simulink model "sldemo_bus_arrays"  (Simulink 10.0)
settings: Solver=FixedStepDiscrete  StartTime=0.0  StopTime=10  FixedStep=0.2  RelTol=1e-3  EnableMultiTasking=on
PreLoadFcn:
  | load sldemo_bus_arrays_data.mat;
undefined symbols (not defined in the file): a, b
Description:
  | Modeling Arrays of Buses
  | 
  | This example illustrates the use of arrays of buses in Simulink(R) to represent structured data compactly, eliminating the need to include multiple copies of the same buses.You can also use For Each subsystems to iteratively process each element of the bus array.
  | 
  | In this example, the array of buses is created using a Vector Concatenate block. The input bus signals to the Concatenate block must be nonvirtual and of the same type (that is, have the same names, hierarchies and attributes for the leaf elements).
  | 
  | The example also illustrates the use of the Selector and Assignment blocks to select from and assign into the array of buses.
CloseFcn:
  | evalin('base', 'clear sldemo_bus_arrays_busobject;');
settings Model: Creator=The MathWorks, Inc.  LastModifiedBy=bhisma
settings DataIOCC: LimitDataPoints=on  SaveFormat=StructureWithTime  SaveOutput=off  SaveTime=off  ReturnWorkspaceOutputs=on
settings OptimizationCC: BlockReduction=off  OptimizeBlockIOStorage=off  BufferReuse=off  GlobalBufferReuse=off  ExpressionFolding=off  PassReuseOutputArgsAs=Individual arguments  ExpressionDepthLimit=2147483647  LocalBlockOutputs=off  EfficientFloat2IntCast=on  OptimizeDataStoreBuffers=off  BusAssignmentInplaceUpdate=off  EfficientTunableParamExpr=on
settings DebuggingCC: ConsistencyChecking=warning  SignalInfNanChecking=error  SignalRangeChecking=error  ReadBeforeWriteMsg=EnableAllAsError  WriteAfterWriteMsg=EnableAllAsError  WriteAfterReadMsg=EnableAllAsError  AlgebraicLoopMsg=error  SaveWithDisabledLinksMsg=error  SaveWithParameterizedLinksMsg=error  UnderspecifiedInitializationDetection=Simplified  MergeDetectMultiDrivingBlocksExec=error  CheckExecutionContextPreStartOutputMsg=on  CheckExecutionContextRuntimeOutputMsg=on  BlockPriorityViolationMsg=error  SolverPrmCheckMsg=error  InheritedTsInSrcMsg=error  SigSpecEnsureSampleTimeMsg=error  CheckMatrixSingularityMsg=error  IntegerOverflowMsg=error  ParameterUnderflowMsg=error  ParameterPrecisionLossMsg=error  ParameterTunabilityLossMsg=error  UnderSpecifiedDataTypeMsg=error  UnnecessaryDatatypeConvMsg=warning  VectorMatrixConversionMsg=error  FcnCallInpInsideContextMsg=warning  SignalLabelMismatchMsg=error  UnconnectedInputMsg=error  UnconnectedOutputMsg=error  UnconnectedLineMsg=error  SFcnCompatibilityMsg=error  BusObjectLabelMismatch=error  RootOutportRequireBusObject=error  AssertControl=DisableAll  ModelReferenceIOMsg=error  ModelReferenceVersionMismatchMessage=error  ModelReferenceIOMismatchMessage=error  UnknownTsInhSupMsg=error  ModelReferenceDataLoggingMessage=error  StateNameClashWarn=warning  StrictBusMsg=ErrorOnBusTreatedAsVector  IntegerSaturationMsg=error
settings SFSimCC: MATLABDynamicMemAlloc=off
settings RTWCC: Description=Real-Time Workshop Embedded Coder  SystemTargetFile=ert.tlc  GenCodeOnly=on  TemplateMakefile=ert_default_tmf  GenerateReport=on  IncludeHyperlinkInReport=on  LaunchReport=on
settings CodeAppCC: ForceParamTrailComments=on  IgnoreCustomStorageClasses=off  MangleLength=4  CustomSymbolStrType=$N$R$M  InternalIdentifier=Classic  ReqsInCode=on
settings ERTTargetCC: MultiwordLength=2048  GenerateSampleERTMain=on  IncludeMdlTerminateFcn=off  GeneratePreprocessorConditionals=Disable all  SuppressErrorStatus=on  SupportAbsoluteTime=off  SupportNonFinite=off  ParenthesesLevel=Maximum  ERTCustomFileTemplate=example_file_process.tlc  PreserveExpressionOrder=on  PreserveIfCondition=on  ConvertIfToSwitch=off  SuppressUnreachableDefaultCases=off
settings ConfigComp: CovExternalEMLEnable=off

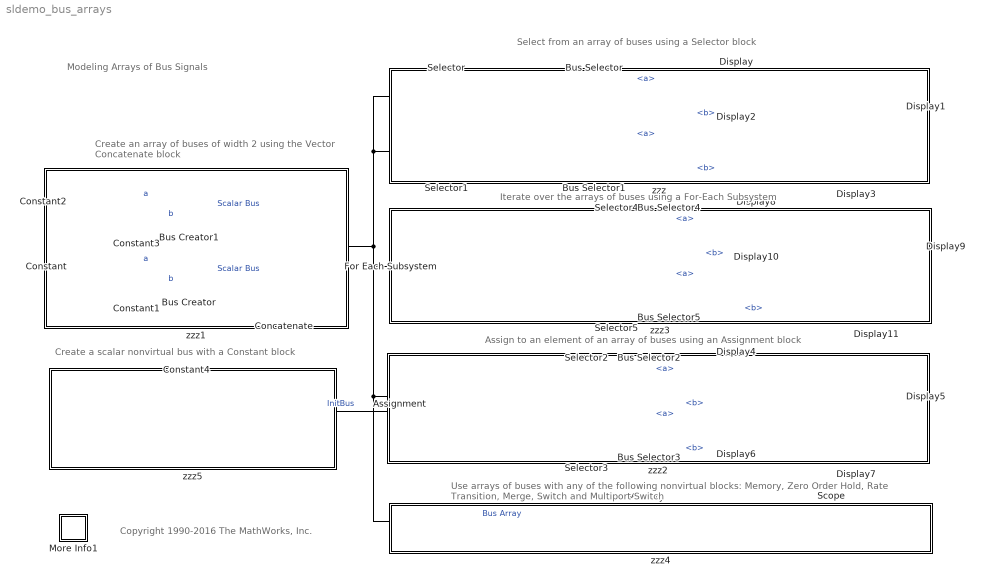
== system sldemo_bus_arrays ==
  note: Copyright 1990-2016 The MathWorks, Inc.
  note: Modeling Arrays of Bus Signals
  note: Select from an array of buses using a Selector block
  note: Create an array of buses of width 2 using
      |  the Vector Concatenate block
  note: Assign to an element of an array of buses using an Assignment block
  note: Iterate over the arrays of buses using a For-Each Subsystem
  note: Use arrays of buses with any of the following nonvirtual blocks:
      | Memory, Zero Order Hold, Rate Transition, Merge, Switch and Multiport Switch
  note: Create a scalar nonvirtual bus with a Constant block
  Assignment : Assignment  IndexOptions=Index vector (dialog)  Indices=1  OutputSizes=1
  Bus Creator : BusCreator  Inputs=2  OutDataTypeStr=Bus: sldemo_bus_arrays_busobject  NonVirtualBus=on
  Bus Creator1 : BusCreator  Inputs=2  OutDataTypeStr=Bus: sldemo_bus_arrays_busobject  NonVirtualBus=on
  Bus Selector{,1..5} (6 alike) : BusSelector  OutputSignals=a,b
  Concatenate : Concatenate
  Constant : Constant  Value=3
  Constant1 : Constant  Value=4
  Constant2 : Constant
  Constant3 : Constant  Value=2
  Constant4 : Constant  Value=struct('a', 0, 'b', -1)  OutDataTypeStr=Bus: sldemo_bus_arrays_busobject
  Display{,1..11} (12 alike) : Display
  For Each Subsystem : Subsystem  TreatAsAtomicUnit=on
  Memory : Memory
  More Info1 : Subsystem
      settings: OpenFcn=showdemo(bdroot(gcs))
      mask Display: disp('?')
  Scope : Scope
  Selector : Selector  InputPortWidth=2  IndexOptions=Index vector (dialog)  Indices=1  OutputSizes=1
  Selector1 : Selector  InputPortWidth=2  IndexOptions=Index vector (dialog)  Indices=2  OutputSizes=1
  Selector2 : Selector  InputPortWidth=2  IndexOptions=Index vector (dialog)  Indices=1  OutputSizes=1
  Selector3 : Selector  InputPortWidth=2  IndexOptions=Index vector (dialog)  Indices=2  OutputSizes=1
  Selector4 : Selector  InputPortWidth=2  IndexOptions=Index vector (dialog)  Indices=1  OutputSizes=1
  Selector5 : Selector  InputPortWidth=2  IndexOptions=Index vector (dialog)  Indices=2  OutputSizes=1
  zzz : Subsystem  TreatAsAtomicUnit=on
      mask Display: disp('')
  zzz1 : Subsystem  TreatAsAtomicUnit=on
      mask Display: disp('')
  zzz2 : Subsystem  TreatAsAtomicUnit=on
      mask Display: disp('')
  zzz3 : Subsystem  TreatAsAtomicUnit=on
      mask Display: disp('')
  zzz4 : Subsystem  TreatAsAtomicUnit=on
      mask Display: disp('')
  zzz5 : Subsystem  TreatAsAtomicUnit=on
      mask Display: disp('')
  wires:
  Constant/1 -> Bus Creator/1  "a"
  Constant1/1 -> Bus Creator/2  "b"
  Constant2/1 -> Bus Creator1/1  "a"
  Constant3/1 -> Bus Creator1/2  "b"
  Bus Creator1/1 -> Concatenate/1  "Scalar Bus"
  Bus Creator/1 -> Concatenate/2  "Scalar Bus"
  Constant4/1 -> Assignment/2  "InitBus"
  Selector/1 -> Bus Selector/1
  Selector1/1 -> Bus Selector1/1
  Bus Selector/1 -> Display/1  "<a>"
  Bus Selector/2 -> Display1/1  "<b>"
  Bus Selector1/1 -> Display2/1  "<a>"
  Bus Selector1/2 -> Display3/1  "<b>"
  Assignment/1 -> Selector3/1, Selector2/1
  Selector2/1 -> Bus Selector2/1
  Bus Selector2/1 -> Display4/1  "<a>"
  Bus Selector2/2 -> Display5/1  "<b>"
  Bus Selector3/1 -> Display6/1  "<a>"
  Bus Selector3/2 -> Display7/1  "<b>"
  Selector3/1 -> Bus Selector3/1
  Selector4/1 -> Bus Selector4/1
  Selector5/1 -> Bus Selector5/1
  Bus Selector4/1 -> Display8/1  "<a>"
  Bus Selector4/2 -> Display9/1  "<b>"
  Bus Selector5/1 -> Display10/1  "<a>"
  Bus Selector5/2 -> Display11/1  "<b>"
  For Each Subsystem/1(Out1) -> Selector4/1, Selector5/1
  Concatenate/1 -> Selector/1, Selector1/1, Memory/1, Assignment/1, For Each Subsystem/1(In1)  "Bus Array"
  Memory/1 -> Scope/1

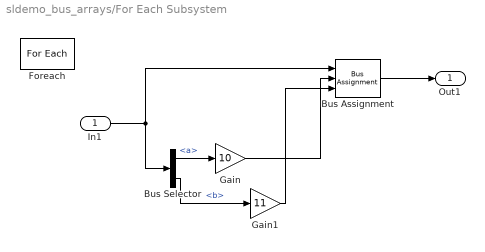
== system sldemo_bus_arrays/For Each Subsystem ==
  In1 : Inport  Partition=on  PartitionDimension=1  PartitionWidth=1  PartitionOffset=0
  Bus Assignment : BusAssignment  AssignedSignals=a,b
  Bus Selector : BusSelector  OutputSignals=a,b
  Foreach : ForEach  DisableCoverage=on
  Gain : Gain  Gain=10
  Gain1 : Gain  Gain=11
  Out1 : Outport  ConcatenationDimension=1  VectorParamsAs1DForOutWhenUnconnected=off
  wires:
  In1/1 -> Bus Selector/1, Bus Assignment/1
  Bus Selector/1 -> Gain/1  "<a>"
  Bus Selector/2 -> Gain1/1  "<b>"
  Gain/1 -> Bus Assignment/2
  Gain1/1 -> Bus Assignment/3
  Bus Assignment/1 -> Out1/1

== system sldemo_bus_arrays/More Info1 ==

== system sldemo_bus_arrays/zzz ==

== system sldemo_bus_arrays/zzz1 ==

== system sldemo_bus_arrays/zzz2 ==

== system sldemo_bus_arrays/zzz3 ==

== system sldemo_bus_arrays/zzz4 ==

== system sldemo_bus_arrays/zzz5 ==
